simulink model "ValidateFloating"  (R2016b)
settings: Solver=FixedStepAuto  StartTime=0.0  StopTime=10.0  RelTol=1e-3
settings Model: Creator=NEATdemo  LastModifiedBy=NEATdemo

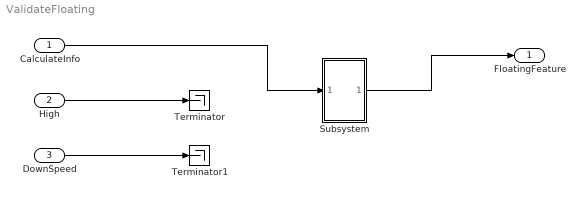
== system ValidateFloating ==
  CalculateInfo : Inport
  High : Inport  Port=2
      settings: AttributesFormatString=Distance
  DownSpeed : Inport  Port=3
      settings: AttributesFormatString=Speed
  Subsystem : Subsystem
  Terminator : Terminator
  Terminator1 : Terminator
  FloatingFeature : Outport
      settings: AttributesFormatString=SystemFeature
  wires:
  High/1 -> Terminator/1
  DownSpeed/1 -> Terminator1/1
  CalculateInfo/1 -> Subsystem/1(In1)
  Subsystem/1(Out1) -> FloatingFeature/1

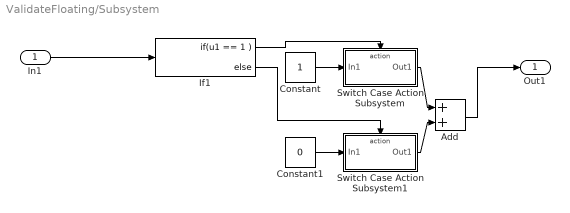
== system ValidateFloating/Subsystem ==
  In1 : Inport
  Add : Sum
  Constant : Constant
  Constant1 : Constant  Value=0
  If1 : If  IfExpression=u1 == 1
  Switch Case Action Subsystem : Subsystem  TreatAsAtomicUnit=on
  Switch Case Action Subsystem1 : Subsystem  TreatAsAtomicUnit=on
  Out1 : Outport
  wires:
  Constant1/1 -> Switch Case Action Subsystem1/1(In1)
  Switch Case Action Subsystem/1(Out1) -> Add/1
  In1/1 -> If1/1
  Constant/1 -> Switch Case Action Subsystem/1(In1)
  Switch Case Action Subsystem1/1(Out1) -> Add/2
  If1/1 -> Switch Case Action Subsystem/Action
  Add/1 -> Out1/1
  If1/2 -> Switch Case Action Subsystem1/Action

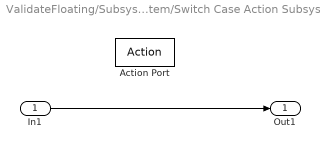
== system ValidateFloating/Subsystem/Switch Case Action Subsystem ==
  In1 : Inport
  Action Port : ActionPort  ActionType=then
  Out1 : Outport
  wires:
  In1/1 -> Out1/1

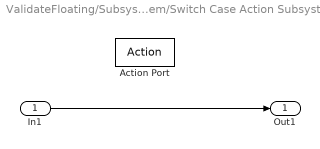
== system ValidateFloating/Subsystem/Switch Case Action Subsystem1 ==
  In1 : Inport
  Action Port : ActionPort  ActionType=else
  Out1 : Outport
  wires:
  In1/1 -> Out1/1
